simulink model "Battery_Thevenin_2RC"  (R2024b)
settings: Solver=ode23t  StartTime=0.0  StopTime=3600  RelTol=1e-4  AbsTol=1e-6
settings Model: Creator=z004f2se  LastModifiedBy=z004f2se

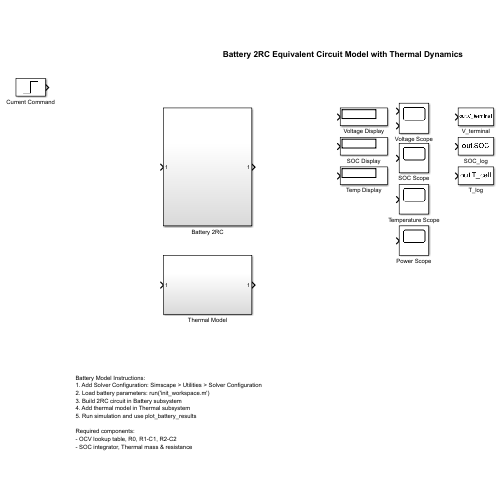
[thumbnail: Simulink's stored preview of the top-level diagram]
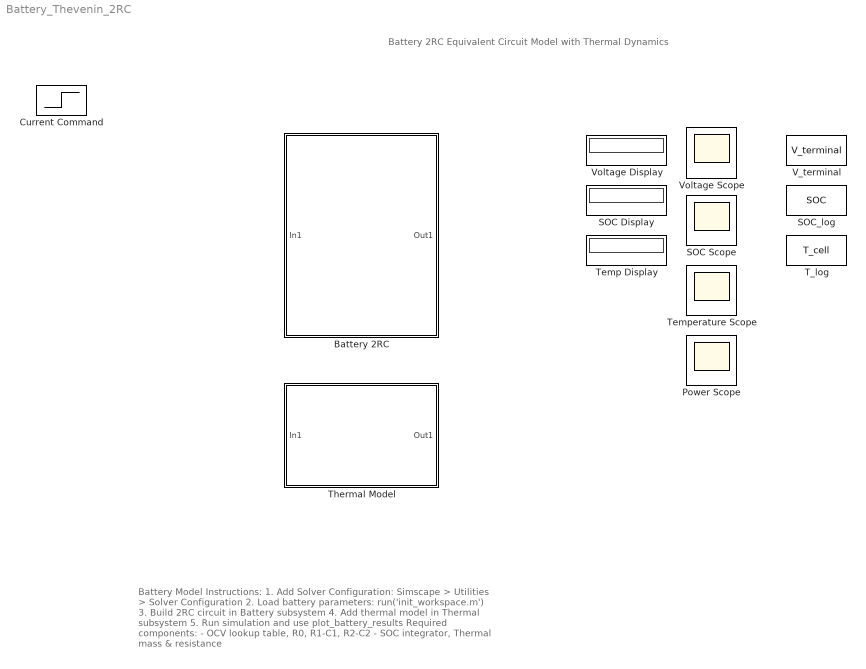
== system Battery_Thevenin_2RC ==
  note: Battery 2RC Equivalent Circuit Model with Thermal Dynamics
  note: Battery Model Instructions:
      | 1. Add Solver Configuration: Simscape > Utilities > Solver Configuration
      | 2. Load battery parameters: run('init_workspace.m')
      | 3. Build 2RC circuit in Battery subsystem
      | 4. Add thermal model in Thermal subsystem
      | 5. Run simulation and use plot_battery_results
      |
      | Required components:
      | - OCV lookup table, R0, R1-C1, R2-C2
      | - SOC integrator, Thermal mass & resistance
  Battery 2RC : Subsystem
  Current Command : Step  Time=10  After=3.5  SampleTime=0
  Power Scope : Scope
  SOC Display : Display
  SOC Scope : Scope
  SOC_log : ToWorkspace  VariableName=SOC  SaveFormat=Timeseries  SampleTime=-1
  T_log : ToWorkspace  VariableName=T_cell  SaveFormat=Timeseries  SampleTime=-1
  Temp Display : Display
  Temperature Scope : Scope
  Thermal Model : Subsystem
  V_terminal : ToWorkspace  VariableName=V_terminal  SaveFormat=Timeseries  SampleTime=-1
  Voltage Display : Display
  Voltage Scope : Scope  NumInputPorts=2

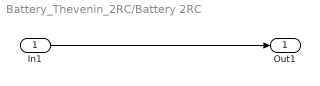
== system Battery_Thevenin_2RC/Battery 2RC ==
  In1 : Inport
  Out1 : Outport
  wires:
  In1/1 -> Out1/1

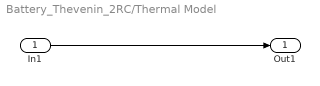
== system Battery_Thevenin_2RC/Thermal Model ==
  In1 : Inport
  Out1 : Outport
  wires:
  In1/1 -> Out1/1
